simulink model "cx06_MA"  (Simulink 7.5)
settings: Solver=FixedStepDiscrete  StartTime=0.0  StopTime=10.0  RelTol=1e-3
undefined symbols (not defined in the file or in its folder): DiscIntNeverNeededParam, ECU555, int, motohawk_build_version, motohawk_trunc_name, motohawk_vardec_path
libraries: MotoHawk_lib x811, simulink x43, simulink_need_slupdate x1
(part 8 of 10)

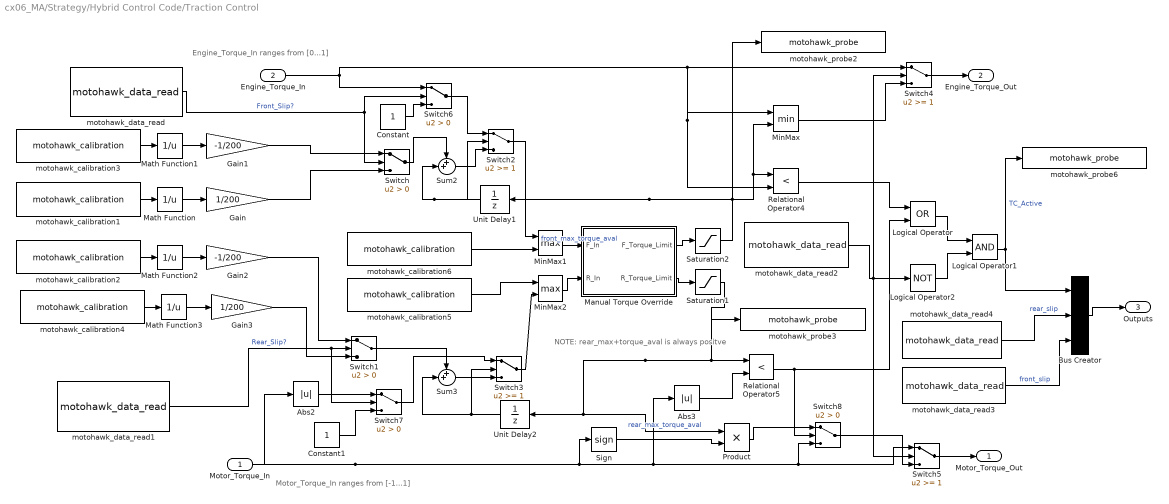
== system cx06_MA/Strategy/Hybrid Control Code/Traction Control ==
  note: Motor_Torque_In
      | ranges from [-1...1]
  note: Engine_Torque_In
      | ranges from [0...1]
  note: NOTE:
      | rear_max+torque_aval
      | is always positve
  Motor_Torque_In : Inport  OutDataType=sfix(16)  OutScaling=2^0
  Engine_Torque_In : Inport  Port=2  OutDataType=sfix(16)  OutScaling=2^0
  Abs2 : Abs
  Abs3 : Abs
  Bus Creator : BusCreator  Inputs=3
  Constant : Constant  OutDataType=sfix(16)  OutScaling=2^0
  Constant1 : Constant  OutDataType=sfix(16)  OutScaling=2^0
  Gain : Gain  Gain=1/200  ParameterDataType=sfix(16)  ParameterScaling=2^0  OutDataType=sfix(16)  OutScaling=2^0
  Gain1 : Gain  Gain=-1/200  ParameterDataType=sfix(16)  ParameterScaling=2^0  OutDataType=sfix(16)  OutScaling=2^0
  Gain2 : Gain  Gain=-1/200  ParameterDataType=sfix(16)  ParameterScaling=2^0  OutDataType=sfix(16)  OutScaling=2^0
  Gain3 : Gain  Gain=1/200  ParameterDataType=sfix(16)  ParameterScaling=2^0  OutDataType=sfix(16)  OutScaling=2^0
  Logical Operator : Logic  Operator=OR  AllPortsSameDT=off  OutDataTypeMode=boolean  OutDataTypeStr=boolean
  Logical Operator1 : Logic  AllPortsSameDT=off  OutDataTypeMode=boolean  OutDataTypeStr=boolean
  Logical Operator2 : Logic  Operator=NOT  AllPortsSameDT=off  OutDataTypeMode=boolean  OutDataTypeStr=boolean
  Manual Torque Override : Subsystem
  Math Function{,1..3} (4 alike) : Math  Operator=reciprocal  OutDataType=sfix(16)  OutScaling=2^0  SaturateOnIntegerOverflow=on
  MinMax : MinMax  Inputs=2  OutDataType=sfix(16)  OutScaling=2^0
  MinMax1 : MinMax  Function=max  Inputs=2  OutDataType=sfix(16)  OutScaling=2^0
  MinMax2 : MinMax  Function=max  Inputs=2  OutDataType=sfix(16)  OutScaling=2^0
  Product : Product  OutDataType=sfix(16)  OutScaling=2^0  RndMeth=Zero
  Relational Operator4 : RelationalOperator  Operator=<  LogicOutDataTypeMode=boolean  OutDataTypeStr=boolean
  Relational Operator5 : RelationalOperator  Operator=<  LogicOutDataTypeMode=Specify via dialog  OutDataTypeStr=uint(8)
  Saturation1 : Saturate  UpperLimit=1  LowerLimit=0
  Saturation2 : Saturate  UpperLimit=1  LowerLimit=0
  Sign : Signum
  Sum2 : Sum  Inputs=++|  OutDataType=sfix(16)  OutScaling=2^0
  Sum3 : Sum  Inputs=++|  OutDataType=sfix(16)  OutScaling=2^0
  Switch{,1,6..8} (5 alike) : Switch  Criteria=u2 > Threshold
  Switch{2..5} (4 alike) : Switch  Threshold=1
  Unit Delay1 : UnitDelay  X0=1  SampleTime=-1
  Unit Delay2 : UnitDelay  X0=1  SampleTime=-1
  motohawk_calibration1 : MotoHawk_lib/Calibration & Probing Blocks/motohawk_calibration  nam='F_rmp_out_rate'  val=8  storage=Calibration  show_more=on  name_source=Use Parameter  data_type=Inherit from 'Default Value'  read_level=1  write_level=1  ovr_cals=on  view_as=Number  enum_struct={'Disabled', 'Enabled'}  vector_style=Wide Row  use_help_units=on  help='time to ramp up max torque available from 0 to 1'  units='sec'  use_header_enum=off  row_header_enum={}  col_header_enum={}  use_min_max=on  min_val=0.001  max_val=inf  use_precision=on  precision='1.4'  gain=1  offset=0  exp=1  use_mototune_group=off  mototune_group=motohawk_vardec_path(gcb)
  motohawk_calibration2 : MotoHawk_lib/Calibration & Probing Blocks/motohawk_calibration  nam='R_rmp_in_rate'  val=3  storage=Calibration  show_more=on  name_source=Use Parameter  data_type=Inherit from 'Default Value'  read_level=1  write_level=1  ovr_cals=on  view_as=Number  enum_struct={'Disabled', 'Enabled'}  vector_style=Wide Row  use_help_units=on  help='time it takes to ramp down max torque available from 1 to 0'  units='sec'  use_header_enum=off  row_header_enum={}  col_header_enum={}  use_min_max=on  min_val=0.001  max_val=inf  use_precision=on  precision='1.4'  gain=1  offset=0  exp=1  use_mototune_group=off  mototune_group=motohawk_vardec_path(gcb)
  motohawk_calibration3 : MotoHawk_lib/Calibration & Probing Blocks/motohawk_calibration  nam='F_rmp_in_rate'  val=3  storage=Calibration  show_more=on  name_source=Use Parameter  data_type=Inherit from 'Default Value'  read_level=1  write_level=1  ovr_cals=on  view_as=Number  enum_struct={'Disabled', 'Enabled'}  vector_style=Wide Row  use_help_units=on  help='time it takes to ramp down max torque available from 1 to 0'  units='sec'  use_header_enum=off  row_header_enum={}  col_header_enum={}  use_min_max=on  min_val=0.001  max_val=inf  use_precision=on  precision='1.4'  gain=1  offset=0  exp=1  use_mototune_group=off  mototune_group=motohawk_vardec_path(gcb)
  motohawk_calibration4 : MotoHawk_lib/Calibration & Probing Blocks/motohawk_calibration  nam='R_rmp_out_rate'  val=6  storage=Calibration  show_more=on  name_source=Use Parameter  data_type=Inherit from 'Default Value'  read_level=1  write_level=1  ovr_cals=on  view_as=Number  enum_struct={'Disabled', 'Enabled'}  vector_style=Wide Row  use_help_units=on  help='time to ramp up max torque available from 0 to 1'  units='sec'  use_header_enum=off  row_header_enum={}  col_header_enum={}  use_min_max=on  min_val=0.001  max_val=inf  use_precision=on  precision='1.4'  gain=1  offset=0  exp=1  use_mototune_group=off  mototune_group=motohawk_vardec_path(gcb)
  motohawk_calibration5 : MotoHawk_lib/Calibration & Probing Blocks/motohawk_calibration  nam='R_low_bound'  val=.2  storage=Calibration  show_more=on  name_source=Use Parameter  data_type=Inherit from 'Default Value'  read_level=1  write_level=1  ovr_cals=on  view_as=Number  enum_struct={'Disabled', 'Enabled'}  vector_style=Wide Row  use_help_units=on  help='Low Bound for Torque Limit to Rear'  units='%'  use_header_enum=off  row_header_enum={}  col_header_enum={}  use_min_max=on  min_val=0  max_val=1  use_precision=on  precision='1.4'  gain=1  offset=0  exp=1  use_mototune_group=off  mototune_group=motohawk_vardec_path(gcb)
  motohawk_calibration6 : MotoHawk_lib/Calibration & Probing Blocks/motohawk_calibration  nam='F_low_bound'  val=.2  storage=Calibration  show_more=on  name_source=Use Parameter  data_type=Inherit from 'Default Value'  read_level=1  write_level=1  ovr_cals=on  view_as=Number  enum_struct={'Disabled', 'Enabled'}  vector_style=Wide Row  use_help_units=on  help='Low Bound for Torque Limit to Front'  units='%'  use_header_enum=off  row_header_enum={}  col_header_enum={}  use_min_max=on  min_val=0  max_val=1  use_precision=on  precision='1.4'  gain=1  offset=0  exp=1  use_mototune_group=off  mototune_group=motohawk_vardec_path(gcb)
  motohawk_data_read : MotoHawk_lib/Data Storage Blocks/motohawk_data_read  source=Lookup By Name  structure=Scalar  operation=Read scalar from location by index  sz_vec=4  sz_row=2  sz_col=3  typ=uint8  nam='TC_Front_Slip'  checkNull=on  struct_inst_name='Struct1'  struct_nam='MyStruct'
  motohawk_data_read1 : MotoHawk_lib/Data Storage Blocks/motohawk_data_read  source=Lookup By Name  structure=Scalar  operation=Read scalar from location by index  sz_vec=4  sz_row=2  sz_col=3  typ=uint8  nam='TC_Rear_Slip'  checkNull=on  struct_inst_name='Struct1'  struct_nam='MyStruct'
  motohawk_data_read2 : MotoHawk_lib/Data Storage Blocks/motohawk_data_read  source=Lookup By Name  structure=Scalar  operation=Read scalar from location by index  sz_vec=4  sz_row=2  sz_col=3  typ=uint8  nam='inhibitTC'  checkNull=on  struct_inst_name='Struct1'  struct_nam='MyStruct'
  motohawk_data_read3 : MotoHawk_lib/Data Storage Blocks/motohawk_data_read  source=Lookup By Name  structure=Scalar  operation=Read scalar from location by index  sz_vec=4  sz_row=2  sz_col=3  typ=uint8  nam='TC_Front_Slip'  checkNull=on  struct_inst_name='Struct1'  struct_nam='MyStruct'
  motohawk_data_read4 : MotoHawk_lib/Data Storage Blocks/motohawk_data_read  source=Lookup By Name  structure=Scalar  operation=Read scalar from location by index  sz_vec=4  sz_row=2  sz_col=3  typ=uint8  nam='TC_Rear_Slip'  checkNull=on  struct_inst_name='Struct1'  struct_nam='MyStruct'
  motohawk_probe2 : MotoHawk_lib/Calibration & Probing Blocks/motohawk_probe  nam='front_max_torque_aval'  show_more=on  name_source=Use Parameter  read_level=1  view_as=Number  enum_struct={'Disabled', 'Enabled'}  vector_style=Wide Row  use_help_units=off  help=''  units=''  use_header_enum=off  row_header_enum={}  col_header_enum={}  use_precision=off  precision=''  gain=1  offset=0  exp=1  use_mototune_group=off  mototune_group=motohawk_vardec_path(gcb)
  motohawk_probe3 : MotoHawk_lib/Calibration & Probing Blocks/motohawk_probe  nam='rear_max_torque_aval'  show_more=on  name_source=Use Parameter  read_level=1  view_as=Number  enum_struct={'Disabled', 'Enabled'}  vector_style=Wide Row  use_help_units=off  help=''  units=''  use_header_enum=off  row_header_enum={}  col_header_enum={}  use_precision=off  precision=''  gain=1  offset=0  exp=1  use_mototune_group=off  mototune_group=motohawk_vardec_path(gcb)
  motohawk_probe6 : MotoHawk_lib/Calibration & Probing Blocks/motohawk_probe  nam='TC_Indictator'  show_more=on  name_source=Use Parameter  read_level=1  view_as=Enumeration  enum_struct={'OFF', 'ON'}  vector_style=Wide Row  use_help_units=off  help=''  units=''  use_header_enum=off  row_header_enum={}  col_header_enum={}  use_precision=off  precision=''  gain=1  offset=0  exp=1  use_mototune_group=off  mototune_group=motohawk_vardec_path(gcb)
  Motor_Torque_Out : Outport  OutDataType=sfix(16)  OutScaling=2^0
  Engine_Torque_Out : Outport  Port=2  OutDataType=sfix(16)  OutScaling=2^0
  Outputs : Outport  Port=3  OutDataType=sfix(16)  OutScaling=2^0
  wires:
  Logical Operator/1 -> Logical Operator1/1
  Logical Operator1/1 -> motohawk_probe6/1, Bus Creator/1  "TC_Active"
  Logical Operator2/1 -> Logical Operator1/2
  Unit Delay1/1 -> Sum2/2, Switch2/2
  Switch/1 -> Sum2/1
  Switch1/1 -> Sum3/1
  Saturation1/1 -> Unit Delay2/1, Product/1, Relational Operator5/1, motohawk_probe3/1  "rear_max_torque_aval"
  Engine_Torque_In/1 -> Switch4/1, MinMax/1, Relational Operator4/2, Switch6/1
  motohawk_calibration1/1 -> Math Function/1
  Gain/1 -> Switch/3
  motohawk_calibration3/1 -> Math Function1/1
  Gain1/1 -> Switch/1
  Unit Delay2/1 -> Sum3/2, Switch3/2
  Motor_Torque_In/1 -> Abs2/1, Switch5/1, Switch8/3, Abs3/1, Sign/1
  MinMax/1 -> Switch4/3
  motohawk_data_read2/1 -> Switch4/2, Logical Operator2/1, Switch5/2
  Switch5/1 -> Motor_Torque_Out/1
  Switch4/1 -> Engine_Torque_Out/1
  Relational Operator4/1 -> Logical Operator/1
  Relational Operator5/1 -> Logical Operator/2, Switch8/2
  Sum2/1 -> Switch2/3
  Switch6/1 -> Switch2/1
  Constant/1 -> Switch6/3
  Constant1/1 -> Switch7/3
  Switch7/1 -> Switch3/1
  Abs2/1 -> Switch7/1
  Abs3/1 -> Relational Operator5/2
  Switch8/1 -> Switch5/3
  Product/1 -> Switch8/1
  Sign/1 -> Product/2
  Math Function1/1 -> Gain1/1
  Math Function/1 -> Gain/1
  Sum3/1 -> Switch3/3
  motohawk_data_read/1 -> Switch/2, Switch6/2  "Front_Slip?"
  motohawk_data_read1/1 -> Switch1/2, Switch7/2  "Rear_Slip?"
  motohawk_calibration2/1 -> Math Function2/1
  Math Function2/1 -> Gain2/1
  Gain2/1 -> Switch1/1
  motohawk_calibration4/1 -> Math Function3/1
  Math Function3/1 -> Gain3/1
  Gain3/1 -> Switch1/3
  Saturation2/1 -> Unit Delay1/1, MinMax/2, Relational Operator4/1, motohawk_probe2/1
  Manual Torque Override/1(F_Torque_Limit) -> Saturation2/1
  Manual Torque Override/2(R_Torque_Limit) -> Saturation1/1
  MinMax1/1 -> Manual Torque Override/1(F_In)  "front_max_torque_aval"
  Switch2/1 -> MinMax1/1
  motohawk_calibration6/1 -> MinMax1/2
  MinMax2/1 -> Manual Torque Override/2(R_In)
  Switch3/1 -> MinMax2/2
  motohawk_calibration5/1 -> MinMax2/1
  Bus Creator/1 -> Outputs/1
  motohawk_data_read4/1 -> Bus Creator/2  "rear_slip"
  motohawk_data_read3/1 -> Bus Creator/3  "front_slip"

== system cx06_MA/Strategy/Hybrid Control Code/ZEV ==
  In1 : Inport  OutDataType=sfix(16)  OutScaling=2^0
  Action Port : ActionPort  ActionType=case
  Bus Creator : BusCreator  Inputs='engine_Torque','motor_Torque','motor_Enable'
  Bus Selector : BusSelector  OutputSignals=Analog.Driver.Accel
  Bus Selector2 : BusSelector  OutputSignals=JCI.SOC
  Constant : Constant  OutDataType=sfix(16)  OutScaling=2^0
  Constant1 : Constant  Value=0  OutDataType=sfix(16)  OutScaling=2^0
  SOC_RampOut : Subsystem
  motohawk_interpolation_1d : MotoHawk_lib/Lookup Tables/motohawk_interpolation_1d  nam='ZEV_Accel_Map'  table_data=[0:0.1:1]  show_more=on  data_type=double  storage=NonAdaptive  read_level=1  write_level=1  ovr_cals=on  use_help=off  help=''  units=''  use_min_max=off  min_val=0  max_val=1  use_precision=off  precision='1.2'  gain=1  offset=0  exp=1  use_links=on  prelookup_block='Diesel_Accel_Ord'  output_name=''  use_mototune_group=off  mototune_group=motohawk_vardec_path(gcb)
  motohawk_prelookup : MotoHawk_lib/Lookup Tables/motohawk_prelookup  nam='ZEV_Accel_Ord'  breakpoint_data=[0:0.1:1]  show_more=on  data_type=double  storage=Constant  read_level=1  write_level=1  ovr_cals=on  use_help=off  help=''  units=''  use_min_max=off  min_val=-inf  max_val=inf  use_precision=off  precision=''  gain=1  offset=0  exp=1  use_links=off  input_name=''  use_mototune_group=off  mototune_group=motohawk_vardec_path(gcb)
  Outputs : Outport  OutDataType=sfix(16)  OutScaling=2^0  InitialOutput=0
  wires:
  Bus Creator/1 -> Outputs/1
  Constant/1 -> Bus Creator/3  "motor_Enable"
  Constant1/1 -> Bus Creator/1  "engine_Torque"
  In1/1 -> Bus Selector/1, Bus Selector2/1
  Bus Selector/1 -> motohawk_prelookup/1  "<Accel>"
  motohawk_prelookup/1 -> motohawk_interpolation_1d/1
  motohawk_interpolation_1d/1 -> SOC_RampOut/1(Torque_In)
  Bus Selector2/1 -> SOC_RampOut/2(SOC)  "<SOC>"
  SOC_RampOut/1(Torque_Out) -> Bus Creator/2  "motor_Torque"

== system cx06_MA/Strategy/Hybrid Control Code/diesel ==
  Inputs : Inport  OutDataType=sfix(16)  OutScaling=2^0
  Action Port : ActionPort  ActionType=case
  Bus Creator : BusCreator  Inputs='engine_Torque','motor_Torque','motor_Enable'
  Bus Selector : BusSelector  OutputSignals=Analog.Driver.Accel
  Constant : Constant  Value=0  OutDataType=sfix(16)  OutScaling=2^0
  Constant1 : Constant  Value=0  OutDataType=sfix(16)  OutScaling=2^0
  motohawk_interpolation_1d : MotoHawk_lib/Lookup Tables/motohawk_interpolation_1d  nam='Diesel_Accel_Map'  table_data=[0:0.1:1]  show_more=on  data_type=double  storage=NonAdaptive  read_level=1  write_level=1  ovr_cals=on  use_help=off  help=''  units=''  use_min_max=off  min_val=0  max_val=1  use_precision=off  precision='1.2'  gain=1  offset=0  exp=1  use_links=on  prelookup_block='Diesel_Accel_Ord'  output_name=''  use_mototune_group=off  mototune_group=motohawk_vardec_path(gcb)
  motohawk_prelookup : MotoHawk_lib/Lookup Tables/motohawk_prelookup  nam='Diesel_Accel_Ord'  breakpoint_data=[0:0.1:1]  show_more=on  data_type=double  storage=Constant  read_level=1  write_level=1  ovr_cals=on  use_help=off  help=''  units=''  use_min_max=off  min_val=-inf  max_val=inf  use_precision=off  precision=''  gain=1  offset=0  exp=1  use_links=off  input_name=''  use_mototune_group=off  mototune_group=motohawk_vardec_path(gcb)
  Outputs : Outport  OutDataType=sfix(16)  OutScaling=2^0  InitialOutput=0
  wires:
  Constant/1 -> Bus Creator/2  "motor_Torque"
  Constant1/1 -> Bus Creator/3  "motor_Enable"
  motohawk_prelookup/1 -> motohawk_interpolation_1d/1
  Bus Creator/1 -> Outputs/1
  motohawk_interpolation_1d/1 -> Bus Creator/1  "engine_Torque"
  Inputs/1 -> Bus Selector/1
  Bus Selector/1 -> motohawk_prelookup/1  "<Accel>"

== system cx06_MA/Strategy/Hybrid Control Code/sustain Brake ==
  Inputs : Inport  OutDataType=sfix(16)  OutScaling=2^0
  "state " : Inport  Port=2  OutDataType=sfix(16)  OutScaling=2^0
  Bus Selector : BusSelector  OutputSignals=JCI.SOC
  Bus Selector1 : BusSelector  OutputSignals=IPT.Status 2.veh_speed
  C4 : simulink/Logic and Bit Operations/Compare To Constant  SystemSampleTime=-1  relop===  const=4  LogicOutDataTypeMode=uint8
  Compare To Zero : simulink/Logic and Bit Operations/Compare To Zero  SystemSampleTime=-1  relop===  LogicOutDataTypeMode=uint8  ZeroCross=off
  Constant : Constant  Value=0  OutDataType=sfix(16)  OutScaling=2^0
  Logical Operator : Logic  Operator=OR  Inputs=3  AllPortsSameDT=off  OutDataTypeMode=boolean  OutDataTypeStr=boolean
  Product : Product  OutDataType=sfix(16)  OutScaling=2^0  RndMeth=Zero
  Sustain Brake original : Stateflow chart  TreatAsAtomicUnit=on
  Switch : Switch  Criteria=u2 > Threshold
  motohawk_calibration1 : MotoHawk_lib/Calibration & Probing Blocks/motohawk_calibration  nam='SB_Off'  val=80  storage=Calibration  show_more=on  name_source=Use Parameter  data_type=Inherit from 'Default Value'  read_level=1  write_level=1  ovr_cals=on  view_as=Number  enum_struct={'Disabled', 'Enabled'}  vector_style=Wide Row  use_help_units=off  help='Above this SOC sustain brake turns off'  units='%'  use_header_enum=off  row_header_enum={}  col_header_enum={}  use_min_max=on  min_val=0  max_val=100  use_precision=off  precision=''  gain=1  offset=0  exp=1  use_mototune_group=off  mototune_group=motohawk_vardec_path(gcb)
  motohawk_calibration2 : MotoHawk_lib/Calibration & Probing Blocks/motohawk_calibration  nam='SB_On'  val=60  storage=Calibration  show_more=on  name_source=Use Parameter  data_type=Inherit from 'Default Value'  read_level=1  write_level=1  ovr_cals=on  view_as=Number  enum_struct={'Disabled', 'Enabled'}  vector_style=Wide Row  use_help_units=off  help='Below this SOC, sustain brake turns on'  units='%'  use_header_enum=off  row_header_enum={}  col_header_enum={}  use_min_max=on  min_val=0  max_val=100  use_precision=off  precision=''  gain=1  offset=0  exp=1  use_mototune_group=off  mototune_group=motohawk_vardec_path(gcb)
  motohawk_calibration3 : MotoHawk_lib/Calibration & Probing Blocks/motohawk_calibration  nam='SB_Ramp_Time'  val=1000  storage=Calibration  show_more=on  name_source=Use Parameter  data_type=double  read_level=1  write_level=1  ovr_cals=on  view_as=Number  enum_struct={'Disabled', 'Enabled'}  vector_style=Wide Row  use_help_units=off  help='SB ramps in over this amount of time'  units='s'  use_header_enum=off  row_header_enum={}  col_header_enum={}  use_min_max=off  min_val=0  max_val=60  use_precision=on  precision=''  gain=0.005  offset=0  exp=1  use_mototune_group=off  mototune_group=motohawk_vardec_path(gcb)
  motohawk_calibration4 : MotoHawk_lib/Calibration & Probing Blocks/motohawk_calibration  nam='SB_Level'  val=-.1  storage=Calibration  show_more=on  name_source=Use Parameter  data_type=single  read_level=1  write_level=1  ovr_cals=on  view_as=Number  enum_struct={'Disabled', 'Enabled'}  vector_style=Wide Row  use_help_units=on  help='Sustain Brake Regen Level'  units='%'  use_header_enum=off  row_header_enum={}  col_header_enum={}  use_min_max=off  min_val=-1  max_val=0  use_precision=on  precision='1.2'  gain=1  offset=0  exp=1  use_mototune_group=off  mototune_group=motohawk_vardec_path(gcb)
  motohawk_data_read : MotoHawk_lib/Data Storage Blocks/motohawk_data_read  source=Lookup By Name  structure=Scalar  operation=Read scalar from location by index  sz_vec=4  sz_row=2  sz_col=3  typ=uint8  nam='inhibitRegen'  checkNull=on  struct_inst_name='Struct1'  struct_nam='MyStruct'
  motohawk_probe : MotoHawk_lib/Calibration & Probing Blocks/motohawk_probe  nam='Sustain_Brake'  show_more=on  name_source=Use Parameter  read_level=1  view_as=Enumeration  enum_struct={'False', 'True'}  vector_style=Wide Row  use_help_units=off  help=''  units=''  use_header_enum=off  row_header_enum={}  col_header_enum={}  use_precision=off  precision=''  gain=1  offset=0  exp=1  use_mototune_group=off  mototune_group=motohawk_vardec_path(gcb)
  motohawk_probe1 : MotoHawk_lib/Calibration & Probing Blocks/motohawk_probe  nam='Sustain_Brake_Level'  show_more=on  name_source=Use Parameter  read_level=1  view_as=Number  enum_struct={'False', 'True'}  vector_style=Wide Row  use_help_units=off  help=''  units=''  use_header_enum=off  row_header_enum={}  col_header_enum={}  use_precision=on  precision='1.3'  gain=1  offset=0  exp=1  use_mototune_group=off  mototune_group=motohawk_vardec_path(gcb)
  speed_RampOut : Subsystem
  Torque_Req : Outport  OutDataType=sfix(16)  OutScaling=2^0
  wires:
  motohawk_calibration4/1 -> Product/1
  Product/1 -> speed_RampOut/1(Torque_In), motohawk_probe1/1
  Bus Selector1/1 -> speed_RampOut/2(speed)  "<veh_speed>"
  speed_RampOut/1(Torque_Out) -> Switch/3
  Switch/1 -> Torque_Req/1
  "state "/1 -> Compare To Zero/1, C4/1
  Compare To Zero/1 -> Logical Operator/1
  Logical Operator/1 -> Switch/2
  Constant/1 -> Switch/1
  Bus Selector/1 -> Sustain Brake original/1(SOC)  "<SOC>"
  motohawk_calibration1/1 -> Sustain Brake original/2(SB_Off)
  motohawk_calibration2/1 -> Sustain Brake original/3(SB_On)
  motohawk_calibration3/1 -> Sustain Brake original/4(ramp_time)
  Sustain Brake original/2(SB) -> motohawk_probe/1
  Sustain Brake original/1(level) -> Product/2
  Inputs/1 -> Bus Selector/1, Bus Selector1/1
  C4/1 -> Logical Operator/2
  motohawk_data_read/1 -> Logical Operator/3

== system cx06_MA/Strategy/Urea Control Code/Dosing_Alg ==
  Engine_Run_Status : Inport  OutDataType=sfix(16)  OutScaling=2^0
  ESS_Req_Eng_Kill : Inport  Port=2  OutDataType=sfix(16)  OutScaling=2^0
  Compare To Constant : simulink/Logic and Bit Operations/Compare To Constant  SystemSampleTime=-1  relop=>=  const=1  LogicOutDataTypeMode=uint8  ZeroCross=off
  Compare To Constant1 : simulink/Logic and Bit Operations/Compare To Constant  SystemSampleTime=-1  relop===  const=1  LogicOutDataTypeMode=uint8  ZeroCross=off
  Constant : Constant  Value=0  OutDataType=sfix(16)  OutScaling=2^0
  Constant1 : Constant  OutDataType=sfix(16)  OutScaling=2^0
  Constant2 : Constant  OutDataType=sfix(16)  OutScaling=2^0
  Constant3 : Constant  Value=0  OutDataType=sfix(16)  OutScaling=2^0
  Data Type Conversion : DataTypeConversion  OutDataTypeMode=uint8  OutDataType=sfix(16)  OutScaling=2^0  OutDataTypeStr=uint8
  Gain1 : Gain  Gain=1/200  ParameterDataType=sfix(16)  ParameterScaling=2^0  OutDataType=sfix(16)  OutScaling=2^0
  Logical Operator : Logic  AllPortsSameDT=off  OutDataTypeMode=boolean  OutDataTypeStr=boolean
  Logical Operator1 : Logic  AllPortsSameDT=off  OutDataTypeMode=boolean  OutDataTypeStr=boolean
  Logical Operator2 : Logic  Operator=NOT  AllPortsSameDT=off  OutDataTypeMode=boolean  OutDataTypeStr=boolean
  Relational Operator1 : RelationalOperator  Operator=<  LogicOutDataTypeMode=Specify via dialog  OutDataTypeStr=uint(8)
  Relational Operator2 : RelationalOperator  Operator=>  LogicOutDataTypeMode=Specify via dialog  OutDataTypeStr=uint(8)
  Saturation : Saturate  UpperLimit=6000  LowerLimit=0
  Sum : Sum  Inputs=|++  OutDataType=sfix(16)  OutScaling=2^0
  Switch1 : Switch  Criteria=u2 > Threshold  OutDataTypeStr=Inherit: Inherit via back propagation
  Switch2 : Switch  Criteria=u2 > Threshold  OutDataTypeStr=Inherit: Inherit via back propagation
  Unit Delay : UnitDelay  X0=1  SampleTime=-1
  motohawk_calibration11 : MotoHawk_lib/Calibration & Probing Blocks/motohawk_calibration  nam='Dose_Freq'  val=5  storage=Calibration  show_more=on  name_source=Use Parameter  data_type=double  read_level=1  write_level=1  ovr_cals=on  view_as=Number  enum_struct={'False', 'True'}  vector_style=Wide Row  use_help_units=off  help=''  units=''  use_header_enum=off  row_header_enum={}  col_header_enum={}  use_min_max=on  min_val=0  max_val=40  use_precision=on  precision='1.1'  gain=1  offset=0  exp=1  use_mototune_group=off  mototune_group=motohawk_vardec_path(gcb)
  motohawk_calibration2 : MotoHawk_lib/Calibration & Probing Blocks/motohawk_calibration  nam='Dosing_Time'  val=200  storage=Calibration  show_more=on  name_source=Use Parameter  data_type=double  read_level=1  write_level=1  ovr_cals=on  view_as=Number  enum_struct={'False', 'True'}  vector_style=Wide Row  use_help_units=on  help='Time to Dose when engine starts'  units='sec'  use_header_enum=off  row_header_enum={}  col_header_enum={}  use_min_max=on  min_val=0  max_val=6000  use_precision=on  precision='1.3'  gain=1/200  offset=0  exp=1  use_mototune_group=off  mototune_group=motohawk_vardec_path(gcb)
  motohawk_probe1 : MotoHawk_lib/Calibration & Probing Blocks/motohawk_probe  nam='Dosing_Cnt'  show_more=off  name_source=Use Parameter  read_level=1  view_as=Number  enum_struct={'Disabled', 'Enabled'}  vector_style=Wide Row  use_help_units=off  help=''  units=''  use_header_enum=off  row_header_enum={}  col_header_enum={}  use_precision=off  precision=''  gain=1  offset=0  exp=1  use_mototune_group=off  mototune_group=motohawk_vardec_path(gcb)
  Dose_Freq : Outport  OutDataType=sfix(16)  OutScaling=2^0
  Urea_OK_Eng_Kill : Outport  Port=2  OutDataType=sfix(16)  OutScaling=2^0
  wires:
  motohawk_calibration2/1 -> Relational Operator1/2
  Switch1/1 -> Saturation/1
  Saturation/1 -> Unit Delay/1, Relational Operator1/1, Relational Operator2/1, Gain1/1
  Unit Delay/1 -> Sum/1
  Constant1/1 -> Sum/2
  Gain1/1 -> motohawk_probe1/1
  Switch2/1 -> Dose_Freq/1
  Data Type Conversion/1 -> Switch2/2
  Constant2/1 -> Relational Operator2/2
  Relational Operator1/1 -> Logical Operator/1, Logical Operator2/1
  Relational Operator2/1 -> Logical Operator/2
  Logical Operator/1 -> Data Type Conversion/1
  motohawk_calibration11/1 -> Switch2/1
  Constant3/1 -> Switch2/3
  Sum/1 -> Switch1/1
  Constant/1 -> Switch1/3
  Engine_Run_Status/1 -> Compare To Constant/1
  ESS_Req_Eng_Kill/1 -> Compare To Constant1/1
  Compare To Constant/1 -> Logical Operator1/1
  Compare To Constant1/1 -> Logical Operator1/2
  Logical Operator1/1 -> Switch1/2
  Logical Operator2/1 -> Urea_OK_Eng_Kill/1

== system cx06_MA/Strategy/Urea Control Code/LeanRich ==
  note: State
      | 1 - Neutral
      | 2 - Lean
      | 3 - Lean2Rich
      | 4 - Rich2Lean
      | 5 - Rich
      | 6 - Error
  Inputs : Inport  OutDataType=sfix(16)  OutScaling=2^0
  Bus Selector : BusSelector  OutputSignals=Urea.NOx_Mid.NOxMid_NOx,Urea.Temperature.Temp_1
  Bus Selector1 : BusSelector  OutputSignals=Urea.NOx_Mid.NoxMid_ECM_Er_Code
  Chart : Stateflow chart  TreatAsAtomicUnit=on
  Compare To Zero : simulink/Logic and Bit Operations/Compare To Zero  SystemSampleTime=-1  relop=~=  LogicOutDataTypeMode=uint8  ZeroCross=off
  Constant : Constant  OutDataType=sfix(16)  OutScaling=2^0
  Logical Operator : Logic  Operator=OR  AllPortsSameDT=off  OutDataTypeMode=boolean  OutDataTypeStr=boolean
  Switch : Switch  Criteria=u2 ~= 0
  motohawk_calibration : MotoHawk_lib/Calibration & Probing Blocks/motohawk_calibration  nam='NOxThres'  val=0  storage=Calibration  show_more=on  name_source=Use Parameter  data_type=Inherit from 'Default Value'  read_level=1  write_level=1  ovr_cals=on  view_as=Number  enum_struct={'Disabled', 'Enabled'}  vector_style=Wide Row  use_help_units=on  help='Threshold level for ammonia present'  units='ppm'  use_header_enum=off  row_header_enum={}  col_header_enum={}  use_min_max=off  min_val=-inf  max_val=inf  use_precision=off  precision=''  gain=1  offset=0  exp=1  use_mototune_group=off  mototune_group=motohawk_vardec_path(gcb)
  motohawk_calibration1 : MotoHawk_lib/Calibration & Probing Blocks/motohawk_calibration  nam='AmmoniaMinTemp'  val=0  storage=Calibration  show_more=on  name_source=Use Parameter  data_type=Inherit from 'Default Value'  read_level=1  write_level=1  ovr_cals=on  view_as=Number  enum_struct={'Disabled', 'Enabled'}  vector_style=Wide Row  use_help_units=on  help='Below this temp Cats not active and ammonia detection disabled'  units='C'  use_header_enum=off  row_header_enum={}  col_header_enum={}  use_min_max=off  min_val=-inf  max_val=inf  use_precision=off  precision=''  gain=1  offset=0  exp=1  use_mototune_group=off  mototune_group=motohawk_vardec_path(gcb)
  motohawk_calibration2 : MotoHawk_lib/Calibration & Probing Blocks/motohawk_calibration  nam='LeanMult'  val=0  storage=Calibration  show_more=on  name_source=Use Parameter  data_type=Inherit from 'Default Value'  read_level=1  write_level=1  ovr_cals=on  view_as=Number  enum_struct={'Disabled', 'Enabled'}  vector_style=Wide Row  use_help_units=on  help='Multiplier to Apply for Lean Operation'  units=''  use_header_enum=off  row_header_enum={}  col_header_enum={}  use_min_max=on  min_val=0  max_val=10  use_precision=off  precision=''  gain=1  offset=0  exp=1  use_mototune_group=off  mototune_group=motohawk_vardec_path(gcb)
  motohawk_calibration3 : MotoHawk_lib/Calibration & Probing Blocks/motohawk_calibration  nam='RichMult'  val=0  storage=Calibration  show_more=on  name_source=Use Parameter  data_type=Inherit from 'Default Value'  read_level=1  write_level=1  ovr_cals=on  view_as=Number  enum_struct={'Disabled', 'Enabled'}  vector_style=Wide Row  use_help_units=on  help='Multiplier to Apply for Rich Operation'  units=''  use_header_enum=off  row_header_enum={}  col_header_enum={}  use_min_max=on  min_val=0  max_val=10  use_precision=off  precision=''  gain=1  offset=0  exp=1  use_mototune_group=off  mototune_group=motohawk_vardec_path(gcb)
  motohawk_calibration4 : MotoHawk_lib/Calibration & Probing Blocks/motohawk_calibration  nam='LeanTime'  val=0  storage=Calibration  show_more=on  name_source=Use Parameter  data_type=Inherit from 'Default Value'  read_level=1  write_level=1  ovr_cals=on  view_as=Number  enum_struct={'Disabled', 'Enabled'}  vector_style=Wide Row  use_help_units=on  help='No Ammonia this long to go Rich'  units='s'  use_header_enum=off  row_header_enum={}  col_header_enum={}  use_min_max=on  min_val=0  max_val=300  use_precision=on  precision=''  gain=0.05  offset=0  exp=1  use_mototune_group=off  mototune_group=motohawk_vardec_path(gcb)
  motohawk_calibration5 : MotoHawk_lib/Calibration & Probing Blocks/motohawk_calibration  nam='RichTime'  val=0  storage=Calibration  show_more=on  name_source=Use Parameter  data_type=Inherit from 'Default Value'  read_level=1  write_level=1  ovr_cals=on  view_as=Number  enum_struct={'Disabled', 'Enabled'}  vector_style=Wide Row  use_help_units=on  help='Ammonia this long to go Lean'  units='s'  use_header_enum=off  row_header_enum={}  col_header_enum={}  use_min_max=on  min_val=0  max_val=300  use_precision=on  precision=''  gain=0.05  offset=0  exp=1  use_mototune_group=off  mototune_group=motohawk_vardec_path(gcb)
  motohawk_calibration6 : MotoHawk_lib/Calibration & Probing Blocks/motohawk_calibration  nam='LeanRichEnable'  val=0  storage=Calibration  show_more=on  name_source=Use Parameter  data_type=uint8  read_level=1  write_level=1  ovr_cals=on  view_as=Enumeration  enum_struct={'Disabled', 'Enabled'}  vector_style=Wide Row  use_help_units=on  help='Enables the Lean/Rich Strategy'  units=''  use_header_enum=off  row_header_enum={}  col_header_enum={}  use_min_max=off  min_val=-inf  max_val=inf  use_precision=on  precision=''  gain=1  offset=0  exp=1  use_mototune_group=off  mototune_group=motohawk_vardec_path(gcb)
  motohawk_fault_action : MotoHawk_lib/Fault Management Blocks/motohawk_fault_action  nam='UreaLeanRich'  output_status=on  eval_nam=UreaLeanRich
  motohawk_probe : MotoHawk_lib/Calibration & Probing Blocks/motohawk_probe  nam='Ammonia'  show_more=on  name_source=Use Parameter  read_level=1  view_as=Enumeration  enum_struct={'False', 'True'}  vector_style=Wide Row  use_help_units=off  help=''  units=''  use_header_enum=off  row_header_enum={}  col_header_enum={}  use_precision=off  precision=''  gain=1  offset=0  exp=1  use_mototune_group=off  mototune_group=motohawk_vardec_path(gcb)
  motohawk_probe1 : MotoHawk_lib/Calibration & Probing Blocks/motohawk_probe  nam='LeanRichMult'  show_more=off  name_source=Use Parameter  read_level=1  view_as=Number  enum_struct={'Disabled', 'Enabled'}  vector_style=Wide Row  use_help_units=off  help=''  units=''  use_header_enum=off  row_header_enum={}  col_header_enum={}  use_precision=off  precision=''  gain=1  offset=0  exp=1  use_mototune_group=off  mototune_group=motohawk_vardec_path(gcb)
  motohawk_probe2 : MotoHawk_lib/Calibration & Probing Blocks/motohawk_probe  nam='LeanRichState'  show_more=on  name_source=Use Parameter  read_level=1  view_as=Enumeration  enum_struct={'Unknown', 'Neutral', 'Lean', 'Lean2Rich', 'Rich2Lean', 'Rich', 'Error'}  vector_style=Wide Row  use_help_units=off  help=''  units=''  use_header_enum=off  row_header_enum={}  col_header_enum={}  use_precision=off  precision=''  gain=1  offset=0  exp=1  use_mototune_group=off  mototune_group=motohawk_vardec_path(gcb)
  motohawk_probe4 : MotoHawk_lib/Calibration & Probing Blocks/motohawk_probe  nam='LeanCnt'  show_more=on  name_source=Use Parameter  read_level=1  view_as=Number  enum_struct={'Disabled', 'Enabled'}  vector_style=Wide Row  use_help_units=off  help=''  units=''  use_header_enum=off  row_header_enum={}  col_header_enum={}  use_precision=on  precision='1.1'  gain=0.05  offset=0  exp=1  use_mototune_group=off  mototune_group=motohawk_vardec_path(gcb)
  motohawk_probe5 : MotoHawk_lib/Calibration & Probing Blocks/motohawk_probe  nam='RichCnt'  show_more=on  name_source=Use Parameter  read_level=1  view_as=Number  enum_struct={'Disabled', 'Enabled'}  vector_style=Wide Row  use_help_units=off  help=''  units=''  use_header_enum=off  row_header_enum={}  col_header_enum={}  use_precision=on  precision='1.1'  gain=0.05  offset=0  exp=1  use_mototune_group=off  mototune_group=motohawk_vardec_path(gcb)
  Multiplier : Outport  OutDataType=sfix(16)  OutScaling=2^0
  wires:
  Inputs/1 -> Bus Selector/1, Bus Selector1/1
  Chart/1(Ammonia) -> motohawk_probe/1
  Chart/2(LeanCnt) -> motohawk_probe4/1
  Chart/3(RichCnt) -> motohawk_probe5/1
  Chart/4(mult) -> motohawk_probe1/1, Switch/1
  Chart/5(State) -> motohawk_probe2/1
  Bus Selector/1 -> Chart/2(NOx)  "<NOxMid_NOx>"
  Bus Selector/2 -> Chart/3(temp)  "<Temp_1>"
  motohawk_calibration2/1 -> Chart/4(LeanMult)
  motohawk_calibration4/1 -> Chart/5(LeanTime)
  motohawk_calibration3/1 -> Chart/6(RichMult)
  motohawk_calibration5/1 -> Chart/7(RichTime)
  motohawk_calibration/1 -> Chart/8(NOxThres)
  motohawk_calibration1/1 -> Chart/9(minTemp)
  Bus Selector1/1 -> Compare To Zero/1  "<NoxMid_ECM_Er_Code>"
  motohawk_fault_action/1 -> Logical Operator/1
  Compare To Zero/1 -> Logical Operator/2
  Logical Operator/1 -> Chart/1(errorIn)
  motohawk_calibration6/1 -> Switch/2
  Constant/1 -> Switch/3
  Switch/1 -> Multiplier/1

== system cx06_MA/Inputs/Analog Inputs/Driver Inputs/Accel ==
  2pt Calibration1_2 : Fcn  Expr=(u[1]-u[2])/(u[3]-u[2])
  2pt Calibration1_3 : Fcn  Expr=(u[1]-u[2])/(u[3]-u[2])
  Abs : Abs
  Average : Fcn  Expr=(u[1]+u[2])/2
  Constant : Constant  Value=0  OutDataType=sfix(16)  OutScaling=2^0
  Data Type Conversion : DataTypeConversion  OutDataTypeMode=single  OutDataType=sfix(16)  OutScaling=2^0  OutDataTypeStr=single
  Data Type Conversion1 : DataTypeConversion  OutDataTypeMode=single  OutDataType=sfix(16)  OutScaling=2^0  OutDataTypeStr=single
  Logical Operator : Logic  Operator=NOT  AllPortsSameDT=off  OutDataTypeMode=boolean  OutDataTypeStr=boolean
  Mux : Mux  Inputs=3
  Mux1 : Mux  Inputs=3
  Mux2 : Mux  Inputs=2
  Range_Detect : Subsystem
  Range_Detect1 : Subsystem
  Relational Operator : RelationalOperator  Operator=<=  LogicOutDataTypeMode=boolean  OutDataTypeStr=boolean
  Saturation : Saturate  UpperLimit=1  LowerLimit=0
  Saturation1 : Saturate  UpperLimit=1  LowerLimit=0
  Sum : Sum  Inputs=+|-  OutDataType=sfix(16)  OutScaling=2^0
  Switch : Switch  Criteria=u2 ~= 0
  motohawk_ain1 : MotoHawk_lib/Analog I//O Blocks/motohawk_ain  res_name=[]  text_resource=AN2M  code_resource=NONE  val_resource=-1  target=ECU555-80  resource_enum_str=(None)=-1,ECUP=53,DRVP=54,XDRP=55,AN1M=56,AN2M=57,AN3M=58,AN4M=59,AN5M=60,AN6M=61,AN7M=62,AN8M=63,AN9M=64,AN10M=65,AN11M=66,AN12M=67,AN13M=68,AN14M=69,AN15M=70,AN16M=71,AN17M=72,AN18M=73,AN19M=74,O2A=90,O2B=91,XDRP_B=92  altref=5V Reference  typ=uint16  num_adc_bits=10  use_stat=on  use_vardec=on  nam='Accel2'  read_level=1  write_level=1  group='I/O Pins | Inputs Config'
  motohawk_ain4 : MotoHawk_lib/Analog I//O Blocks/motohawk_ain  res_name=[]  text_resource=AN1M  code_resource=NONE  val_resource=-1  target=ECU555-80  resource_enum_str=(None)=-1,ECUP=53,DRVP=54,XDRP=55,AN1M=56,AN2M=57,AN3M=58,AN4M=59,AN5M=60,AN6M=61,AN7M=62,AN8M=63,AN9M=64,AN10M=65,AN11M=66,AN12M=67,AN13M=68,AN14M=69,AN15M=70,AN16M=71,AN17M=72,AN18M=73,AN19M=74,O2A=90,O2B=91,XDRP_B=92  altref=5V Reference  typ=uint16  num_adc_bits=10  use_stat=on  use_vardec=on  nam='Accel1'  read_level=1  write_level=1  group='I/O Pins | Inputs Config'
  motohawk_calibration : MotoHawk_lib/Calibration & Probing Blocks/motohawk_calibration  nam='Accel1_Zero'  val=94  storage=Calibration  show_more=on  name_source=Use Parameter  data_type=Inherit via back propagation  read_level=1  write_level=1  ovr_cals=on  view_as=Number  enum_struct={'Disabled', 'Enabled'}  vector_style=Wide Row  use_help_units=off  help=''  units=''  use_header_enum=off  row_header_enum={}  col_header_enum={}  use_min_max=off  min_val=-inf  max_val=inf  use_precision=off  precision=''  gain=1  offset=0  exp=1  use_mototune_group=off  mototune_group=motohawk_vardec_path(gcb)
  motohawk_calibration1 : MotoHawk_lib/Calibration & Probing Blocks/motohawk_calibration  nam='Accel1_Full'  val=430  storage=Calibration  show_more=on  name_source=Use Parameter  data_type=Inherit via back propagation  read_level=1  write_level=1  ovr_cals=on  view_as=Number  enum_struct={'Disabled', 'Enabled'}  vector_style=Wide Row  use_help_units=off  help=''  units=''  use_header_enum=off  row_header_enum={}  col_header_enum={}  use_min_max=off  min_val=-inf  max_val=inf  use_precision=off  precision=''  gain=1  offset=0  exp=1  use_mototune_group=off  mototune_group=motohawk_vardec_path(gcb)
  motohawk_calibration2 : MotoHawk_lib/Calibration & Probing Blocks/motohawk_calibration  nam='Accel2_Zero'  val=193  storage=Calibration  show_more=on  name_source=Use Parameter  data_type=Inherit via back propagation  read_level=1  write_level=1  ovr_cals=on  view_as=Number  enum_struct={'Disabled', 'Enabled'}  vector_style=Wide Row  use_help_units=off  help=''  units=''  use_header_enum=off  row_header_enum={}  col_header_enum={}  use_min_max=off  min_val=-inf  max_val=inf  use_precision=off  precision=''  gain=1  offset=0  exp=1  use_mototune_group=off  mototune_group=motohawk_vardec_path(gcb)
  motohawk_calibration3 : MotoHawk_lib/Calibration & Probing Blocks/motohawk_calibration  nam='Accel2_Full'  val=865  storage=Calibration  show_more=on  name_source=Use Parameter  data_type=Inherit via back propagation  read_level=1  write_level=1  ovr_cals=on  view_as=Number  enum_struct={'Disabled', 'Enabled'}  vector_style=Wide Row  use_help_units=off  help=''  units=''  use_header_enum=off  row_header_enum={}  col_header_enum={}  use_min_max=off  min_val=-inf  max_val=inf  use_precision=off  precision=''  gain=1  offset=0  exp=1  use_mototune_group=off  mototune_group=motohawk_vardec_path(gcb)
  motohawk_calibration4 : MotoHawk_lib/Calibration & Probing Blocks/motohawk_calibration  nam='Acell_Max_Diff'  val=0.08  storage=Calibration  show_more=on  name_source=Use Parameter  data_type=Inherit from 'Default Value'  read_level=1  write_level=1  ovr_cals=on  view_as=Number  enum_struct={'Disabled', 'Enabled'}  vector_style=Wide Row  use_help_units=on  help='2 Accel pots must be this close together'  units=''  use_header_enum=off  row_header_enum={}  col_header_enum={}  use_min_max=off  min_val=-inf  max_val=inf  use_precision=off  precision=''  gain=1  offset=0  exp=1  use_mototune_group=off  mototune_group=motohawk_vardec_path(gcb)
  motohawk_fault_def : MotoHawk_lib/Fault Management Blocks/motohawk_fault_def  nam='Accel1Range'  mode=Disabled  id=[]  x=10  y=20  input_suspected=on  indeterminate=off  increment_xy=on  downsample_count=1  ovr_cals=on  ovr_actions=on  show_actions=on  action1_name=''  action1_cond=(None)  action2_name=''  action2_cond=(None)  action3_name=''  action3_cond=(None)  action4_name=''  action4_cond=(None)
  motohawk_fault_def1 : MotoHawk_lib/Fault Management Blocks/motohawk_fault_def  nam='Accel2Range'  mode=Disabled  id=[]  x=10  y=20  input_suspected=on  indeterminate=off  increment_xy=on  downsample_count=1  ovr_cals=on  ovr_actions=on  show_actions=on  action1_name=''  action1_cond=(None)  action2_name=''  action2_cond=(None)  action3_name=''  action3_cond=(None)  action4_name=''  action4_cond=(None)
  motohawk_fault_def2 : MotoHawk_lib/Fault Management Blocks/motohawk_fault_def  nam='Accel12Sync'  mode=Disabled  id=[]  x=10  y=20  input_suspected=on  indeterminate=off  increment_xy=on  downsample_count=1  ovr_cals=on  ovr_actions=on  show_actions=on  action1_name='inhibitDiesel'  action1_cond=Active  action2_name='inhibitEV'  action2_cond=Active  action3_name=''  action3_cond=(None)  action4_name=''  action4_cond=(None)
  motohawk_probe : MotoHawk_lib/Calibration & Probing Blocks/motohawk_probe  nam='raw_Accel1'  show_more=on  name_source=Use Parameter  read_level=1  view_as=Number  enum_struct={'Disabled', 'Enabled'}  vector_style=Wide Row  use_help_units=off  help=''  units=''  use_header_enum=off  row_header_enum={}  col_header_enum={}  use_precision=off  precision=''  gain=1  offset=0  exp=1  use_mototune_group=off  mototune_group=motohawk_vardec_path(gcb)
  motohawk_probe1 : MotoHawk_lib/Calibration & Probing Blocks/motohawk_probe  nam='raw_Accel2'  show_more=on  name_source=Use Parameter  read_level=1  view_as=Number  enum_struct={'Disabled', 'Enabled'}  vector_style=Wide Row  use_help_units=off  help=''  units=''  use_header_enum=off  row_header_enum={}  col_header_enum={}  use_precision=off  precision=''  gain=1  offset=0  exp=1  use_mototune_group=off  mototune_group=motohawk_vardec_path(gcb)
  motohawk_probe10 : MotoHawk_lib/Calibration & Probing Blocks/motohawk_probe  nam='In_Accel2'  show_more=on  name_source=Use Parameter  read_level=1  view_as=Number  enum_struct={'Disabled', 'Enabled'}  vector_style=Wide Row  use_help_units=off  help=''  units=''  use_header_enum=off  row_header_enum={}  col_header_enum={}  use_precision=off  precision=''  gain=1  offset=0  exp=1  use_mototune_group=on  mototune_group='Debug | Inputs'
  motohawk_probe2 : MotoHawk_lib/Calibration & Probing Blocks/motohawk_probe  nam='cal_Accel1'  show_more=on  name_source=Use Parameter  read_level=1  view_as=Number  enum_struct={'Disabled', 'Enabled'}  vector_style=Wide Row  use_help_units=off  help=''  units=''  use_header_enum=off  row_header_enum={}  col_header_enum={}  use_precision=off  precision=''  gain=1  offset=0  exp=1  use_mototune_group=off  mototune_group=motohawk_vardec_path(gcb)
  motohawk_probe3 : MotoHawk_lib/Calibration & Probing Blocks/motohawk_probe  nam='cal_Accel2'  show_more=on  name_source=Use Parameter  read_level=1  view_as=Number  enum_struct={'Disabled', 'Enabled'}  vector_style=Wide Row  use_help_units=off  help=''  units=''  use_header_enum=off  row_header_enum={}  col_header_enum={}  use_precision=off  precision=''  gain=1  offset=0  exp=1  use_mototune_group=off  mototune_group=motohawk_vardec_path(gcb)
  motohawk_probe4 : MotoHawk_lib/Calibration & Probing Blocks/motohawk_probe  nam='cal_Accel'  show_more=on  name_source=Use Parameter  read_level=1  view_as=Number  enum_struct={'Disabled', 'Enabled'}  vector_style=Wide Row  use_help_units=off  help=''  units=''  use_header_enum=off  row_header_enum={}  col_header_enum={}  use_precision=on  precision='1.2'  gain=1  offset=0  exp=1  use_mototune_group=off  mototune_group=motohawk_vardec_path(gcb)
  motohawk_probe9 : MotoHawk_lib/Calibration & Probing Blocks/motohawk_probe  nam='In_Accel1'  show_more=on  name_source=Use Parameter  read_level=1  view_as=Number  enum_struct={'Disabled', 'Enabled'}  vector_style=Wide Row  use_help_units=off  help=''  units=''  use_header_enum=off  row_header_enum={}  col_header_enum={}  use_precision=off  precision=''  gain=1  offset=0  exp=1  use_mototune_group=on  mototune_group='Debug | Inputs'
  Accel : Outport  OutDataType=sfix(16)  OutScaling=2^0
  wires:
  motohawk_ain4/1 -> Data Type Conversion/1, motohawk_probe/1
  motohawk_calibration/1 -> Mux/2, Range_Detect/2(Zero)
  motohawk_calibration1/1 -> Mux/3, Range_Detect/3(Full)
  Mux/1 -> 2pt Calibration1_2/1
  2pt Calibration1_2/1 -> Saturation/1
  motohawk_calibration2/1 -> Mux1/2, Range_Detect1/2(Zero)
  motohawk_calibration3/1 -> Mux1/3, Range_Detect1/3(Full)
  Mux1/1 -> 2pt Calibration1_3/1
  2pt Calibration1_3/1 -> Saturation1/1
  motohawk_ain1/1 -> Data Type Conversion1/1, motohawk_probe1/1
  Saturation/1 -> motohawk_probe2/1, Sum/1, Mux2/1
  Saturation1/1 -> Sum/2, motohawk_probe3/1, Mux2/2
  Sum/1 -> Abs/1
  Abs/1 -> Relational Operator/1
  motohawk_calibration4/1 -> Relational Operator/2
  Relational Operator/1 -> Switch/2, Logical Operator/1
  Constant/1 -> Switch/3
  Mux2/1 -> Average/1
  Average/1 -> Switch/1
  Data Type Conversion/1 -> Mux/1, Range_Detect/1(Value)
  Data Type Conversion1/1 -> Mux1/1, Range_Detect1/1(Value)
  Switch/1 -> motohawk_probe4/1, Accel/1  "Accel"
  Range_Detect/1(Fault) -> motohawk_fault_def/1
  Range_Detect1/1(Fault) -> motohawk_fault_def1/1
  Logical Operator/1 -> motohawk_fault_def2/1
  motohawk_ain4/2 -> motohawk_probe9/1
  motohawk_ain1/2 -> motohawk_probe10/1
